simulink model "Tipo3_v4"  (R2018b)
(part 2 of 6)

  Distributed Parameters Line9 : powerlib/Elements/Distributed Parameters Line  Phases=3  Frequency=60  Resistance=[19.10e-3 204.4e-3]  Inductance=[0.818e-3 2.17e-3]  Capacitance=[14.2e-9 9e-9]  Length=23.9  x1=[-0.000106 7.26947372143105e-06 0 0;-0.000104 7.26911967487621e-06 0 0;-0.000102 7.26876149590544e-06 0 0;-0.0001 7.26839918472236e-06 0 0;-9.8e-05 7.26803274153294e-06 0 0;-9.6e-05 7.26766216654549e-06 0 0;-9.4e-05 7.2672874599707e-06 0 0;-9.2e-05 7.26690862202157e-06 0 0;-9e-05 7.26652565291346e-06 0 0;-8.8e-05 7.2661385528641e-06 0 0;-8.6e-05 7.26574732209355e-06 0 0;-8.4e-05 7.2653519608242e-06 0 0;-8.2e-05 7.26495246928083e-06 278651.73714618 -560617.530293633;-8e-05 7.26454884769055e-06 279074.353560397 -560407.272500956;-7.8e-05 7.26414109628279e-06 279496.811323862 -560196.696122805;-7.6e-05 7.26372921528938e-06 279919.110196412 -559985.80127889;-7.4e-05 7.26331320494445e-06 280341.249937974 -559774.588089102;-7.2e-05 7.26289306548451e-06 280763.230308568 -559563.056673514;-7e-05 7.26246879714839e-06 281185.051068301 -559351.207152379;-6.8e-05 7.2620404001773e-06 281606.711977373 -559139.039646132;-6.6e-05 7.26160787481476e-06 282028.212796074 -558926.554275386;-6.4e-05 7.26117122130667e-06 282449.553284787 -558713.751160938;-6.2e-05 7.26073043990126e-06 282870.733203982 -558500.630423765;-6e-05 7.26028553084911e-06 283291.752314224 -558287.192185022;-5.8e-05 7.25983649440314e-06 283712.610376169 -558073.436566048;-5.6e-05 7.25938333081863e-06 284133.307150563 -557859.363688359;-5.4e-05 7.2589260403532e-06 284553.842398243 -557644.973673655;-5.2e-05 7.2584646232668e-06 284974.215880142 -557430.266643813;-5e-05 7.25799907982176e-06 285394.42735728 -557215.242720892;-4.8e-05 7.25752941028272e-06 285814.476590772 -556999.902027132;-4.6e-05 7.25705561491669e-06 286234.363341825 -556784.244684949;-4.4e-05 7.25657769399302e-06 286654.087371738 -556568.270816945;-4.2e-05 7.2560956477834e-06 287073.648441902 -556351.980545897;-4e-05 7.25560947656186e-06 287493.046313801 -556135.373994764;-3.8e-05 7.2551191806048e-06 287912.280749011 -555918.451286685;-3.6e-05 7.25462476019093e-06 288331.351509204 -555701.212544978;-3.4e-05 7.25412621560134e-06 288750.258356141 -555483.65789314;-3.2e-05 7.25362354711943e-06 289169.001051679 -555265.78745485;-3e-05 7.25311675503097e-06 289587.579357766 -555047.601353963;-2.8e-05 7.25260583962407e-06 290005.993036446 -554829.099714518;-2.6e-05 7.25209080118918e-06 290424.241849855 -554610.282660729;-2.4e-05 7.25157164001908e-06 290842.325560222 -554391.150316991;-2.2e-05 7.25104835640892e-06 291260.243929873 -554171.702807879;-2e-05 7.25052095065619e-06 291677.996721225 -553951.940258147;-1.8e-05 7.24998942306069e-06 292095.583696789 -553731.862792726;-1.6e-05 7.2494537739246e-06 292513.004619173 -553511.47053673;-1.4e-05 7.24891400355243e-06 292930.259251077 -553290.763615448;-1.2e-05 7.24837011225104e-06 293347.347355295 -553069.742154349;-1e-05 7.24782210032962e-06 293764.268694719 -552848.406279083;-8e-06 7.24726996809971e-06 294181.023032333 -552626.756115476;-6e-06 7.24671371587519e-06 294597.610131217 -552404.791789534;-4e-06 7.24615334397228e-06 295014.029754544 -552182.513427441;-2e-06 7.24558885270956e-06 295430.281665586 -551959.921155561]  x2=[-0.000106 7.70814810497661e-06 0 0;-0.000104 7.70778201230703e-06 0 0;-0.000102 7.70741153784673e-06 0 0;-0.0001 7.70703668180631e-06 0 0;-9.8e-05 7.70665744439887e-06 0 0;-9.6e-05 7.70627382584001e-06 0 0;-9.4e-05 7.70588582634782e-06 0 0;-9.2e-05 7.70549344614285e-06 0 0;-9e-05 7.70509668544819e-06 0 0;-8.8e-05 7.70469554448938e-06 0 0;-8.6e-05 7.70429002349447e-06 0 0;-8.4e-05 7.70388012269399e-06 0 0;-8.2e-05 7.70346584232096e-06 278867.669795074 -561215.499611965;-8e-05 7.7030471826109e-06 279290.737006115 -561005.078839953;-7.8e-05 7.70262414380182e-06 279713.645443392 -560794.33914262;-7.6e-05 7.7021967261342e-06 280136.394866487 -560583.280639769;-7.4e-05 7.70176492985103e-06 280558.98503507 -560371.903451385;-7.2e-05 7.70132875519778e-06 280981.415708903 -560160.207697633;-7e-05 7.70088820242241e-06 281403.686647841 -559948.193498861;-6.8e-05 7.70044327177538e-06 281825.797611825 -559735.860975595;-6.6e-05 7.6999939635096e-06 282247.748360891 -559523.210248545;-6.4e-05 7.69954027788053e-06 282669.538655164 -559310.2414386;-6.2e-05 7.69908221514606e-06 283091.168254861 -559096.954666832;-6e-05 7.69861977556661e-06 283512.636920291 -558883.35005449;-5.8e-05 7.69815295940507e-06 283933.944411851 -558669.427723007;-5.6e-05 7.69768176692681e-06 284355.090490035 -558455.187793996;-5.4e-05 7.69720619839971e-06 284776.074915425 -558240.630389249;-5.2e-05 7.69672625409411e-06 285196.897448695 -558025.75563074;-5e-05 7.69624193428286e-06 285617.557850613 -557810.563640624;-4.8e-05 7.6957532392413e-06 286038.055882038 -557595.054541234;-4.6e-05 7.69526016924725e-06 286458.391303921 -557379.228455085;-4.4e-05 7.69476272458099e-06 286878.563877307 -557163.085504871;-4.2e-05 7.69426090552534e-06 287298.573363331 -556946.625813469;-4e-05 7.69375471236556e-06 287718.419523222 -556729.849503932;-3.8e-05 7.69324414538942e-06 288138.102118304 -556512.756699496;-3.6e-05 7.69272920488718e-06 288557.62090999 -556295.347523575;-3.4e-05 7.69220989115157e-06 288976.975659789 -556077.622099765;-3.2e-05 7.69168620447781e-06 289396.166129302 -555859.58055184;-3e-05 7.69115814516362e-06 289815.192080224 -555641.223003754;-2.8e-05 7.6906257135092e-06 290234.053274343 -555422.549579641;-2.6e-05 7.69008890981721e-06 290652.749473542 -555203.560403815;-2.4e-05 7.68954773439284e-06 291071.280439795 -554984.255600768;-2.2e-05 7.68900218754373e-06 291489.645935173 -554764.635295173;-2e-05 7.68845226958002e-06 291907.845721839 -554544.699611882;-1.8e-05 7.68789798081434e-06 292325.879562051 -554324.448675926;-1.6e-05 7.68733932156179e-06 292743.747218162 -554103.882612515;-1.4e-05 7.68677629213995e-06 293161.448452618 -553883.001547038;-1.2e-05 7.68620889286892e-06 293578.983027961 -553661.805605065;-1e-05 7.68563712407125e-06 293996.350706826 -553440.294912342;-8e-06 7.68506098607197e-06 294413.551251946 -553218.469594795;-6e-06 7.68448047919864e-06 294830.584426145 -552996.329778532;-4e-06 7.68389560378124e-06 295247.449992344 -552773.875589834;-2e-06 7.68330636015228e-06 295664.147713562 -552551.107155165]  x3=[-0.000106 2.0717743763165e-08 0 0;-0.000104 2.07329563718267e-08 0 0;-0.000102 2.07481571940268e-08 0 0;-0.0001 2.07633462211239e-08 0 0;-9.8e-05 2.07785234444833e-08 0 0;-9.6e-05 2.07936888554767e-08 0 0;-9.4e-05 2.08088424454829e-08 0 0;-9.2e-05 2.08239842058871e-08 0 0;-9e-05 2.08391141280815e-08 0 0;-8.8e-05 2.08542322034649e-08 0 0;-8.6e-05 2.08693384234428e-08 0 0;-8.4e-05 2.08844327794274e-08 0 0;-8.2e-05 2.08995152628379e-08 1044.55204684006 -2384.436588464;-8e-05 2.09145858650999e-08 1046.34957259407 -2383.6483370866;-7.8e-05 2.0929644577646e-08 1048.14650350966 -2382.8587306309;-7.6e-05 2.09446913919155e-08 1049.9428385653 -2382.06776954577;-7.4e-05 2.09597262993544e-08 1051.73857673979 -2381.27545428087;-7.2e-05 2.09747492914155e-08 1053.53371701227 -2380.48178528663;-7e-05 2.09897603595585e-08 1055.32825836223 -2379.68676301424;-6.8e-05 2.10047594952497e-08 1057.12219976948 -2378.89038791565;-6.6e-05 2.10197466899623e-08 1058.9155402142 -2378.0926604436;-6.4e-05 2.10347219351762e-08 1060.70827867687 -2377.29358105159;-6.2e-05 2.10496852223781e-08 1062.50041413837 -2376.49315019388;-6e-05 2.10646365430615e-08 1064.29194557986 -2375.69136832552;-5.8e-05 2.10795758887269e-08 1066.0828719829 -2374.88823590231;-5.6e-05 2.10945032508813e-08 1067.87319232935 -2374.08375338081;-5.4e-05 2.11094186210388e-08 1069.66290560143 -2373.27792121837;-5.2e-05 2.112432199072e-08 1071.45201078173 -2372.47073987309;-5e-05 2.11392133514526e-08 1073.24050685314 -2371.66220980386;-4.8e-05 2.1154092694771e-08 1075.02839279892 -2370.8523314703;-4.6e-05 2.11689600122164e-08 1076.81566760269 -2370.04110533283;-4.4e-05 2.1183815295337e-08 1078.6023302484 -2369.22853185262;-4.2e-05 2.11986585356876e-08 1080.38837972035 -2368.41461149161;-4e-05 2.12134897248301e-08 1082.17381500318 -2367.5993447125;-3.8e-05 2.12283088543331e-08 1083.9586350819 -2366.78273197877;-3.6e-05 2.12431159157721e-08 1085.74283894186 -2365.96477375465;-3.4e-05 2.12579109007293e-08 1087.52642556876 -2365.14547050514;-3.2e-05 2.12726938007941e-08 1089.30939394865 -2364.324822696;-3e-05 2.12874646075625e-08 1091.09174306792 -2363.50283079377;-2.8e-05 2.13022233126375e-08 1092.87347191333 -2362.67949526574;-2.6e-05 2.13169699076288e-08 1094.654579472 -2361.85481657996;-2.4e-05 2.13317043841533e-08 1096.43506473137 -2361.02879520526;-2.2e-05 2.13464267338345e-08 1098.21492667926 -2360.20143161122;-2e-05 2.13611369483029e-08 1099.99416430385 -2359.37272626818;-1.8e-05 2.1375835019196e-08 1101.77277659364 -2358.54267964727;-1.6e-05 2.1390520938158e-08 1103.55076253753 -2357.71129222035;-1.4e-05 2.14051946968401e-08 1105.32812112474 -2356.87856446005;-1.2e-05 2.14198562869006e-08 1107.10485134487 -2356.04449683977;-1e-05 2.14345057000043e-08 1108.88095218786 -2355.20908983367;-8e-06 2.14491429278233e-08 1110.65642264402 -2354.37234391668;-6e-06 2.14637679620366e-08 1112.43126170402 -2353.53425956446;-4e-06 2.14783807943298e-08 1114.20546835887 -2352.69483725347;-2e-06 2.14929814163958e-08 1115.97904159996 -2351.85407746091]  x4=[-0.000106 9.5984619497846e-09 0 0;-0.000104 9.58225006844101e-09 0 0;-0.000102 9.56603273969188e-09 0 0;-0.0001 9.54980997275658e-09 0 0;-9.8e-05 9.53358177685757e-09 0 0;-9.6e-05 9.51734816122042e-09 0 0;-9.4e-05 9.50110913507375e-09 0 0;-9.2e-05 9.48486470764927e-09 0 0;-9e-05 9.46861488818178e-09 0 0;-8.8e-05 9.4523596859091e-09 0 0;-8.6e-05 9.43609911007216e-09 0 0;-8.4e-05 9.41983316991492e-09 0 0;-8.2e-05 9.40356187468437e-09 1203.31784535784 -2318.61081330467;-8e-05 9.38728523363058e-09 1205.06569452305 -2317.70287405734;-7.8e-05 9.37100325600665e-09 1206.81285862145 -2316.793617221;-7.6e-05 9.3547159510687e-09 1208.55933665979 -2315.88304331254;-7.4e-05 9.33842332807589e-09 1210.30512764521 -2314.97115284961;-7.2e-05 9.32212539629039e-09 1212.05023058526 -2314.05794635061;-7e-05 9.30582216497741e-09 1213.79464448785 -2313.14342433469;-6.8e-05 9.28951364340516e-09 1215.53836836132 -2312.22758732175;-6.6e-05 9.27319984084486e-09 1217.28140121437 -2311.31043583242;-6.4e-05 9.25688076657072e-09 1219.0237420561 -2310.39197038811;-6.2e-05 9.24055642985996e-09 1220.76538989602 -2309.47219151095;-6e-05 9.2242268399928e-09 1222.50634374402 -2308.55109972382;-5.8e-05 9.20789200625242e-09 1224.24660261038 -2307.62869555035;-5.6e-05 9.191551937925e-09 1225.98616550578 -2306.70497951492;-5.4e-05 9.1752066442997e-09 1227.7250314413 -2305.77995214266;-5.2e-05 9.15885613466864e-09 1229.46319942842 -2304.85361395942;-5e-05 9.14250041832691e-09 1231.20066847901 -2303.92596549183;-4.8e-05 9.12613950457254e-09 1232.93743760533 -2302.99700726724;-4.6e-05 9.10977340270656e-09 1234.67350582005 -2302.06673981376;-4.4e-05 9.0934021220329e-09 1236.40887213623 -2301.13516366023;-4.2e-05 9.07702567185847e-09 1238.14353556734 -2300.20227933624;-4e-05 9.0606440614931e-09 1239.87749512724 -2299.26808737212;-3.8e-05 9.04425730024955e-09 1241.61074983018 -2298.33258829897;-3.6e-05 9.02786539744353e-09 1243.34329869085 -2297.39578264858;-3.4e-05 9.01146836239365e-09 1245.07514072429 -2296.45767095354;-3.2e-05 8.99506620442146e-09 1246.80627494598 -2295.51825374715;-3e-05 8.97865893285139e-09 1248.53670037178 -2294.57753156345;-2.8e-05 8.96224655701081e-09 1250.26641601797 -2293.63550493724;-2.6e-05 8.94582908622998e-09 1251.99542090122 -2292.69217440404;-2.4e-05 8.92940652984205e-09 1253.72371403862 -2291.74754050014;-2.2e-05 8.91297889718305e-09 1255.45129444763 -2290.80160376253;-2e-05 8.89654619759194e-09 1257.17816114617 -2289.85436472899;-1.8e-05 8.88010844041052e-09 1258.90431315251 -2288.90582393801;-1.6e-05 8.86366563498347e-09 1260.62974948537 -2287.95598192881;-1.4e-05 8.84721779065836e-09 1262.35446916384 -2287.00483924138;-1.2e-05 8.8307649167856e-09 1264.07847120745 -2286.05239641643;-1e-05 8.81430702271847e-09 1265.80175463612 -2285.09865399541;-8e-06 8.79784411781312e-09 1267.52431847017 -2284.14361252052;-6e-06 8.78137621142852e-09 1269.24616173036 -2283.18727253468;-4e-06 8.7649033129265e-09 1270.96728343783 -2282.22963458156;-2e-06 8.74842543167173e-09 1272.68768261415 -2281.27069920558]  x5=0.000105620695415245  V1=[1.535e-06 6.231e+05 6.231e+05;377 377 377;-0.6978 0.4703 -1.101]  V2=[1.626e-06 6.236e+05 6.236e+05;377 377 377;-0.6993 0.4702 -1.101]  I1=[6.034e-09 2593 2593;377 377 377;-1.529 0.4282 -1.143]  I2=[4.912e-09 2596 2596;377 377 377;0.3811 0.4816 -1.089]  nHarmo=1  Measurements=None
      settings: SourceProductName=Simscape Power Systems
  Divide : Product  Inputs=*/
  Divide1 : Product  Inputs=*/
  Fourier{,1..3} (4 alike) : powerlib_meascontrol/Measurements/Fourier  Freq=60  n=1  InInit=[0, 0]  Ts=Ts
      settings: SourceProductName=Simscape Power Systems
  Ground : powerlib/Elements/Ground  LConnTagsString=a
  MW1 : Gain  Gain=1/4500  SaturateOnIntegerOverflow=on  OutDataTypeStr=Inherit: Same as input  ParamDataTypeStr=Inherit: Same as input
  MW2 : Gain  Gain=1/400  SaturateOnIntegerOverflow=on  OutDataTypeStr=Inherit: Same as input  ParamDataTypeStr=Inherit: Same as input
  MW3 : Gain  Gain=1/4500  SaturateOnIntegerOverflow=on  OutDataTypeStr=Inherit: Same as input  ParamDataTypeStr=Inherit: Same as input
  MW4 : Gain  Gain=1/400  SaturateOnIntegerOverflow=on  OutDataTypeStr=Inherit: Same as input  ParamDataTypeStr=Inherit: Same as input
  MW5 : Gain  Gain=147*1.5/0.9  SaturateOnIntegerOverflow=on  OutDataTypeStr=Inherit: Same as input  ParamDataTypeStr=Inherit: Same as input
  Mux{1..6} (6 alike) : Mux  Inputs=2
  Polar to Cartesian : simulink_extras/Transformations/Polar to Cartesian
      settings: SourceProductName=Simulink  SourceProductBaseCode=SL
  Polar to Cartesian1 : simulink_extras/Transformations/Polar to Cartesian
      settings: SourceProductName=Simulink  SourceProductBaseCode=SL
  Scope{1,3,10,12} (4 alike) : Scope  NumInputPorts=2
  Scope{5..9,11,13} (7 alike) : Scope
  Sequence Analyzer{,1..3} (4 alike) : powerlib_meascontrol/Measurements/Sequence Analyzer  Freq=60  n=1  seq=Positive Negative Zero  InInit=[1, 0]  Ts=Ts
      settings: SourceProductName=Simscape Power Systems  SourceProductBaseCode=PS
  Subsystem1 : Subsystem  mask{Tini_FT=50.1, Tini_FF=900, Tini_FFT=900, Tini_FFF=900, R_falta=1e-9}
      mask prompts: Tini_FT "Tempo Inicial FT:"; Tini_FF "Tempo Inicial FF:"; Tini_FFT "Tempo Inicial FFT:"; Tini_FFF "Tempo Inicial FFF:"; R_falta "Resist. Falta:"
  Subsystem10 : Subsystem  mask{Tini_FT=50.1, Tini_FF=900, Tini_FFT=900, Tini_FFF=900, R_falta=1e-9}
      mask prompts: Tini_FT "Tempo Inicial FT:"; Tini_FF "Tempo Inicial FF:"; Tini_FFT "Tempo Inicial FFT:"; Tini_FFF "Tempo Inicial FFF:"; R_falta "Resist. Falta:"
  Subsystem11 : Subsystem  mask{Tini_FT=50.1, Tini_FF=900, Tini_FFT=900, Tini_FFF=900, R_falta=1e-9}
      mask prompts: Tini_FT "Tempo Inicial FT:"; Tini_FF "Tempo Inicial FF:"; Tini_FFT "Tempo Inicial FFT:"; Tini_FFF "Tempo Inicial FFF:"; R_falta "Resist. Falta:"
  Subsystem2 : Subsystem  mask{Tini_FT=50.1, Tini_FF=900, Tini_FFT=900, Tini_FFF=900, R_falta=1e-9}
      mask prompts: Tini_FT "Tempo Inicial FT:"; Tini_FF "Tempo Inicial FF:"; Tini_FFT "Tempo Inicial FFT:"; Tini_FFF "Tempo Inicial FFF:"; R_falta "Resist. Falta:"
  Subsystem3 : Subsystem  mask{Tini_FT=50.1, Tini_FF=900, Tini_FFT=900, Tini_FFF=900, R_falta=1e-9}
      mask prompts: Tini_FT "Tempo Inicial FT:"; Tini_FF "Tempo Inicial FF:"; Tini_FFT "Tempo Inicial FFT:"; Tini_FFF "Tempo Inicial FFF:"; R_falta "Resist. Falta:"
  Subsystem4 : Subsystem  mask{Tini_FT=50.1, Tini_FF=900, Tini_FFT=900, Tini_FFF=900, R_falta=1e-9}
      mask prompts: Tini_FT "Tempo Inicial FT:"; Tini_FF "Tempo Inicial FF:"; Tini_FFT "Tempo Inicial FFT:"; Tini_FFF "Tempo Inicial FFF:"; R_falta "Resist. Falta:"
  Subsystem5 : Subsystem  mask{Tini_FT=50.1, Tini_FF=900, Tini_FFT=900, Tini_FFF=900, R_falta=1e-9}
      mask prompts: Tini_FT "Tempo Inicial FT:"; Tini_FF "Tempo Inicial FF:"; Tini_FFT "Tempo Inicial FFT:"; Tini_FFF "Tempo Inicial FFF:"; R_falta "Resist. Falta:"
  Subsystem6 : Subsystem  mask{Tini_FT=50.1, Tini_FF=900, Tini_FFT=900, Tini_FFF=900, R_falta=1e-9}
      mask prompts: Tini_FT "Tempo Inicial FT:"; Tini_FF "Tempo Inicial FF:"; Tini_FFT "Tempo Inicial FFT:"; Tini_FFF "Tempo Inicial FFF:"; R_falta "Resist. Falta:"
  Subsystem7 : Subsystem  mask{Tini_FT=50.1, Tini_FF=900, Tini_FFT=900, Tini_FFF=900, R_falta=1e-9}
      mask prompts: Tini_FT "Tempo Inicial FT:"; Tini_FF "Tempo Inicial FF:"; Tini_FFT "Tempo Inicial FFT:"; Tini_FFF "Tempo Inicial FFF:"; R_falta "Resist. Falta:"
  Subsystem8 : Subsystem  mask{Tini_FT=50.1, Tini_FF=900, Tini_FFT=900, Tini_FFF=900, R_falta=1e-9}
      mask prompts: Tini_FT "Tempo Inicial FT:"; Tini_FF "Tempo Inicial FF:"; Tini_FFT "Tempo Inicial FFT:"; Tini_FFF "Tempo Inicial FFF:"; R_falta "Resist. Falta:"
  Subsystem9 : Subsystem  mask{Tini_FT=50.1, Tini_FF=900, Tini_FFT=900, Tini_FFF=900, R_falta=1e-9}
      mask prompts: Tini_FT "Tempo Inicial FT:"; Tini_FF "Tempo Inicial FF:"; Tini_FFT "Tempo Inicial FFT:"; Tini_FFF "Tempo Inicial FFF:"; R_falta "Resist. Falta:"
  Subtract : Sum  Inputs=+-
  Subtract1 : Sum  Inputs=+-
  Terminal Local : powerlib/Measurements/Three-Phase V-I Measurement  VoltageMeasurement=phase-to-ground  SetLabelV=off  LabelV=Vabc_B120  Vpu=off  VpuLL=off  CurrentMeasurement=yes  SetLabelI=off  LabelI=Iabc_B120  Ipu=off  Pbase=100e6  Vbase=120e3  OutputType=Complex  PhasorSimulation=off  PSBequivalent=0
      settings: SourceProductName=Simscape Electrical
  Terminal Remoto : powerlib/Measurements/Three-Phase V-I Measurement  VoltageMeasurement=phase-to-ground  SetLabelV=off  LabelV=Vabc_B120  Vpu=off  VpuLL=off  CurrentMeasurement=yes  SetLabelI=off  LabelI=Iabc_B120  Ipu=off  Pbase=100e6  Vbase=120e3  OutputType=Complex  PhasorSimulation=off  PSBequivalent=0
      settings: SourceProductName=Simscape Electrical
  Three-Phase Series RLC Branch : powerlib/Elements/Three-Phase Series RLC Branch  LConnTagsString=A|B|C  RConnTagsString=A|B|C  BranchType=RL  Resistance=(500e3^2/10e9)/10  Inductance=(500e3^2/10e9)/377  Capacitance=0  Measurements=None
  Three-Phase Series RLC Branch1 : powerlib/Elements/Three-Phase Series RLC Branch  LConnTagsString=A|B|C  RConnTagsString=A|B|C  BranchType=RL  Resistance=0.191366666666667*18  Inductance=0.002053833333333*18  Capacitance=0  Measurements=None
  Three-Phase Series RLC Branch2 : powerlib/Elements/Three-Phase Series RLC Branch  LConnTagsString=A|B|C  RConnTagsString=A|B|C  BranchType=RL  Resistance=0.214533333333333*1.37  Inductance=0.001806666666667*1.37  Capacitance=0  Measurements=None
  powergui : powerlib/powergui  SimulationMode=Discrete  SampleTime=Ts  frequency=60  Iterations=50  frequencyindice=60  Pbase=100e6  ErrMax=1e-4  UnitsV=kV  UnitsW=MW  buscounter=0  FunctionMessages=off  echomessages=off  EnableUseOfTLC=off  CurrentSourceSwitches=off  DisableSnubberDevices=off  DisableRonSwitches=off  DisableVfSwitches=off  DisplayEquations=off  SolverType=Tustin/Backward Euler (TBE)  Interpol=off  ExternalGateDelay=off  methode=off  Ts=100  x0status=blocks  SPID=off  SwTol=0  HookPort=off  RestoreLinks=warning  ResistiveCurrentMeasurement=off  Frange=[0:0.1:90]  Ylog=off  Xlog=off  ShowGrid=off  save=on  variable=ZData  structure=Vabc_Iabc  ZoomFFT=on  StartTime=0.0  cycles=1  DisplayStyle=1  fundamental=60  FreqAxis=off  MaxFrequency=1000  frequencyindicesteady=1  RmsSteady=1  display=off
  wires:
  Terminal Remoto/1 -> MW3/1
  MW1/1 -> [V_Local]
  [P50] -> Subsystem11/1(In1)
  [P80] -> Subsystem9/1(In1)
  [P90] -> Subsystem8/1(In1)
  [P40] -> Subsystem7/1(In1)
  [P20] -> Subsystem3/1(In1)
  [P30] -> Subsystem4/1(In1)
  [P10] -> Subsystem2/1(In1)
  [P70] -> Subsystem5/1(In1)
  [P60] -> Subsystem6/1(In1)
  [P100] -> Subsystem10/1(In1)
  MW2/1 -> [I_Local]
  MW3/1 -> [V_Remoto]
  MW4/1 -> [I_Remoto]
  Terminal Remoto/2 -> MW4/1
  Compare To Constant6/1 -> [P60]
  Compare To Constant3/1 -> [P30]
  Constant1/1 -> Compare To Constant6/1, Compare To Constant7/1, Compare To Constant8/1, Compare To Constant3/1, Compare To Constant9/1, Compare To Constant10/1, Compare To Constant5/1, Compare To Constant4/1, Compare To Constant2/1, Compare To Constant1/1, Compare To Constant/1
  Compare To Constant1/1 -> [P10]
  Compare To Constant2/1 -> [P20]
  Compare To Constant8/1 -> [P80]
  Compare To Constant7/1 -> [P70]
  Compare To Constant9/1 -> [P90]
  Compare To Constant5/1 -> [P50]
  Compare To Constant/1 -> [P0]
  Compare To Constant10/1 -> [P100]
  Compare To Constant4/1 -> [P40]
  MW5/1 -> Demux1/1
  [P_pu] -> Mux1/1
  Mux1/1 -> MW5/1
  [I_Remoto] -> Demux7/1, Scope1/2, Demux3/1, Sequence Analyzer1/1
  [V_Remoto] -> Demux6/1, Scope1/1, Demux2/1, Sequence Analyzer/1
  [V_Local] -> Demux8/1, Demux4/1, Sequence Analyzer2/1, Scope3/1
  Demux1/2 -> Mux2/2  "Q (Mvar)"
  Demux1/1 -> Mux2/1  "P (MW)"
  [Q_pu] -> Mux1/2
  Mux2/1 -> Scope5/1
  [I_Local] -> Demux9/1, Scope3/2, Demux5/1, Sequence Analyzer3/1
  Constant4/1 -> DFIG Wind Turbine/2(Qref_pu)
  Constant/1 -> DFIG Wind Turbine/1("Wind (m/s) ")
  [P0] -> Subsystem1/1(In1)
  DFIG Wind Turbine/1(m) -> Bus Selector1/1
  Bus Selector1/2 -> [wr]  "<wr_pu (IG speed)>"
  Bus Selector1/4 -> [Q_pu]  "<Q_pu>"
  Bus Selector1/1 -> [Vdc]  "<Vdc_V>"
  Bus Selector1/3 -> [P_pu]  "<P_pu>"
  Sequence Analyzer/2 -> Mux3/2
  Sequence Analyzer/1 -> Mux3/1
  Mux3/1 -> Scope6/1
  Mux4/1 -> Scope7/1
  Sequence Analyzer1/1 -> Mux4/1
  Sequence Analyzer1/2 -> Mux4/2
  Sequence Analyzer3/1 -> Mux6/1
  Mux5/1 -> Scope8/1
  Mux6/1 -> Scope9/1
  Sequence Analyzer2/1 -> Mux5/1
  Sequence Analyzer2/2 -> Mux5/2
  Sequence Analyzer3/2 -> Mux6/2
  Demux2/1 -> Fourier/1  "P (MW)"
  Demux3/1 -> Fourier1/1  "P (MW)"
  Fourier/1 -> Divide/1
  Fourier1/1 -> Divide/2
  Fourier/2 -> Subtract/1
  Fourier1/2 -> Subtract/2
  Demux4/1 -> Fourier2/1  "P (MW)"
  Fourier3/1 -> Divide1/2
  Fourier2/1 -> Divide1/1
  Demux5/1 -> Fourier3/1  "P (MW)"
  Fourier2/2 -> Subtract1/1
  Fourier3/2 -> Subtract1/2
  Demux6/1 -> Scope10/1  "P (MW)"
  Demux7/1 -> Scope10/2, Scope11/1  "P (MW)"
  Demux9/1 -> Scope12/2, Scope13/1  "P (MW)"
  Demux8/1 -> Scope12/1  "P (MW)"
  Divide/1 -> Polar to Cartesian/1
  Divide1/1 -> Polar to Cartesian1/1
  Polar to Cartesian/1 -> Display/1
  Polar to Cartesian/2 -> Display1/1
  Polar to Cartesian1/1 -> Display2/1
  Polar to Cartesian1/2 -> Display3/1
  Terminal Local/1 -> MW1/1
  Terminal Local/2 -> MW2/1
  Subtract/1 -> Degrees to Radians/1
  Degrees to Radians/1 -> Polar to Cartesian/2
  Subtract1/1 -> Degrees to Radians1/1
  Degrees to Radians1/1 -> Polar to Cartesian1/2
  connections:
  Distributed Parameters Line4/RConn3 -- Distributed Parameters Line5/LConn3 -- Subsystem11/RConn3
  Distributed Parameters Line/LConn3 -- Subsystem1/RConn3 -- Terminal Remoto/RConn3
  Distributed Parameters Line/LConn2 -- Subsystem1/RConn2 -- Terminal Remoto/RConn2
  Subsystem10/RConn2 -- Terminal Local/RConn2 -- Distributed Parameters Line9/RConn2
  Distributed Parameters Line9/LConn1 -- Subsystem8/RConn1 -- Distributed Parameters Line8/RConn1
  Distributed Parameters Line7/RConn2 -- Subsystem9/RConn2 -- Distributed Parameters Line8/LConn2
  Distributed Parameters Line9/LConn3 -- Subsystem8/RConn3 -- Distributed Parameters Line8/RConn3
  Distributed Parameters Line6/LConn1 -- Subsystem6/RConn1 -- Distributed Parameters Line5/RConn1
  Distributed Parameters Line5/LConn1 -- Subsystem11/RConn1 -- Distributed Parameters Line4/RConn1
  Distributed Parameters Line2/LConn1 -- Subsystem3/RConn1 -- Distributed Parameters Line1/RConn1
  Distributed Parameters Line9/LConn2 -- Subsystem8/RConn2 -- Distributed Parameters Line8/RConn2
  Subsystem10/RConn3 -- Terminal Local/RConn3 -- Distributed Parameters Line9/RConn3
  Distributed Parameters Line2/RConn3 -- Subsystem4/RConn3 -- Distributed Parameters Line3/LConn3
  Subsystem10/RConn1 -- Terminal Local/RConn1 -- Distributed Parameters Line9/RConn1
  Distributed Parameters Line6/LConn2 -- Subsystem6/RConn2 -- Distributed Parameters Line5/RConn2
  Distributed Parameters Line2/RConn1 -- Subsystem4/RConn1 -- Distributed Parameters Line3/LConn1
  Distributed Parameters Line7/LConn3 -- Subsystem5/RConn3 -- Distributed Parameters Line6/RConn3
  Distributed Parameters Line2/LConn3 -- Subsystem3/RConn3 -- Distributed Parameters Line1/RConn3
  Distributed Parameters Line6/LConn3 -- Subsystem6/RConn3 -- Distributed Parameters Line5/RConn3
  Distributed Parameters Line2/RConn2 -- Subsystem4/RConn2 -- Distributed Parameters Line3/LConn2
  Distributed Parameters Line5/LConn2 -- Subsystem11/RConn2 -- Distributed Parameters Line4/RConn2
  Distributed Parameters Line1/LConn2 -- Subsystem2/RConn2 -- Distributed Parameters Line/RConn2
  Distributed Parameters Line/LConn1 -- Subsystem1/RConn1 -- Terminal Remoto/RConn1
  Distributed Parameters Line7/LConn1 -- Subsystem5/RConn1 -- Distributed Parameters Line6/RConn1
  Distributed Parameters Line1/LConn1 -- Subsystem2/RConn1 -- Distributed Parameters Line/RConn1
  Distributed Parameters Line7/RConn3 -- Subsystem9/RConn3 -- Distributed Parameters Line8/LConn3
  Distributed Parameters Line2/LConn2 -- Subsystem3/RConn2 -- Distributed Parameters Line1/RConn2
  Distributed Parameters Line1/LConn3 -- Subsystem2/RConn3 -- Distributed Parameters Line/RConn3
  Distributed Parameters Line4/LConn3 -- Subsystem7/RConn3 -- Distributed Parameters Line3/RConn3
  Distributed Parameters Line4/LConn1 -- Subsystem7/RConn1 -- Distributed Parameters Line3/RConn1
  Distributed Parameters Line7/LConn2 -- Subsystem5/RConn2 -- Distributed Parameters Line6/RConn2
  Distributed Parameters Line4/LConn2 -- Subsystem7/RConn2 -- Distributed Parameters Line3/RConn2
  Distributed Parameters Line7/RConn1 -- Subsystem9/RConn1 -- Distributed Parameters Line8/LConn1
  Three-Phase Series RLC Branch2/LConn3 -- "138 kV/34,5 kV "/RConn3
  Three-Phase Series RLC Branch/LConn2 -- 500 kV/RConn2
  Three-Phase Series RLC Branch/LConn3 -- 500 kV/RConn3
  Three-Phase Series RLC Branch2/LConn1 -- "138 kV/34,5 kV "/RConn1
  Three-Phase Series RLC Branch2/RConn1 -- 34,5 kV/0,575 kV/LConn1
  Three-Phase Series RLC Branch/LConn1 -- 500 kV/RConn1
  Three-Phase Series RLC Branch1/RConn2 -- "138 kV/34,5 kV "/LConn2
  Three-Phase Series RLC Branch2/LConn2 -- "138 kV/34,5 kV "/RConn2
  Three-Phase Series RLC Branch1/LConn2 -- "500 kV/138 kV "/RConn2
  Three-Phase Series RLC Branch1/LConn1 -- "500 kV/138 kV "/RConn1
  Three-Phase Series RLC Branch/RConn2 -- Terminal Remoto/LConn2
  Terminal Remoto/LConn3 -- Three-Phase Series RLC Branch/RConn3
  Three-Phase Series RLC Branch1/RConn1 -- "138 kV/34,5 kV "/LConn1
  Three-Phase Series RLC Branch2/RConn3 -- 34,5 kV/0,575 kV/LConn3
  Three-Phase Series RLC Branch1/LConn3 -- "500 kV/138 kV "/RConn3
  Three-Phase Series RLC Branch2/RConn2 -- 34,5 kV/0,575 kV/LConn2
  Three-Phase Series RLC Branch1/RConn3 -- "138 kV/34,5 kV "/LConn3
  Terminal Remoto/LConn1 -- Three-Phase Series RLC Branch/RConn1
  Ground/LConn1 -- 500 kV/LConn1
  DFIG Wind Turbine/LConn2 -- 34,5 kV/0,575 kV/RConn2
  DFIG Wind Turbine/LConn1 -- 34,5 kV/0,575 kV/RConn1
  DFIG Wind Turbine/LConn3 -- 34,5 kV/0,575 kV/RConn3
  Terminal Local/LConn3 -- "500 kV/138 kV "/LConn3
  "500 kV/138 kV "/LConn2 -- Terminal Local/LConn2
  Terminal Local/LConn1 -- "500 kV/138 kV "/LConn1
